simulink model "ley_de_control_no_lineal_MGNLC"  (R2023b)
settings: Solver=VariableStepAuto  StartTime=0.0  StopTime=10.0  FixedStep=1e-5  RelTol=1e-3
values from neighbouring files (symbols this model uses):
  L_d = 6.6    [main.m]    (also in parametros.m = 0.0066)
  L_q = 5.8e-3    (= 0.0058)    [diagrama_polos_y_ceros_LTI.m]    (also in main.m = 5.8; parametros.m; variacion_de_parametros.m)
  P_p = 3    [diagrama_polos_y_ceros_LTI.m]    (also in main.m; parametros.m; variacion_de_parametros.m)
settings Model: Creator=nicol  LastModifiedBy=Julya
settings ModelReferenceCC: ModelReferenceMinAlgLoopOccurrences=on

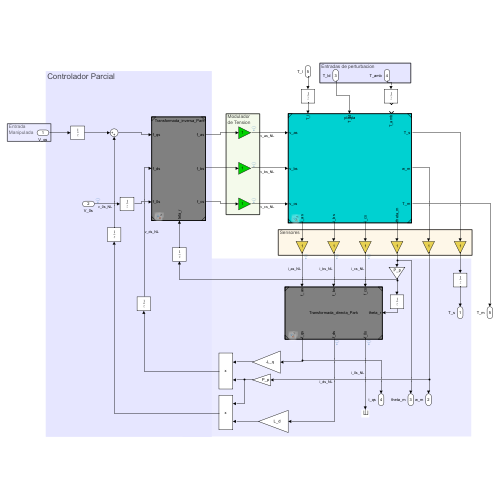
[thumbnail: Simulink's stored preview of the top-level diagram]
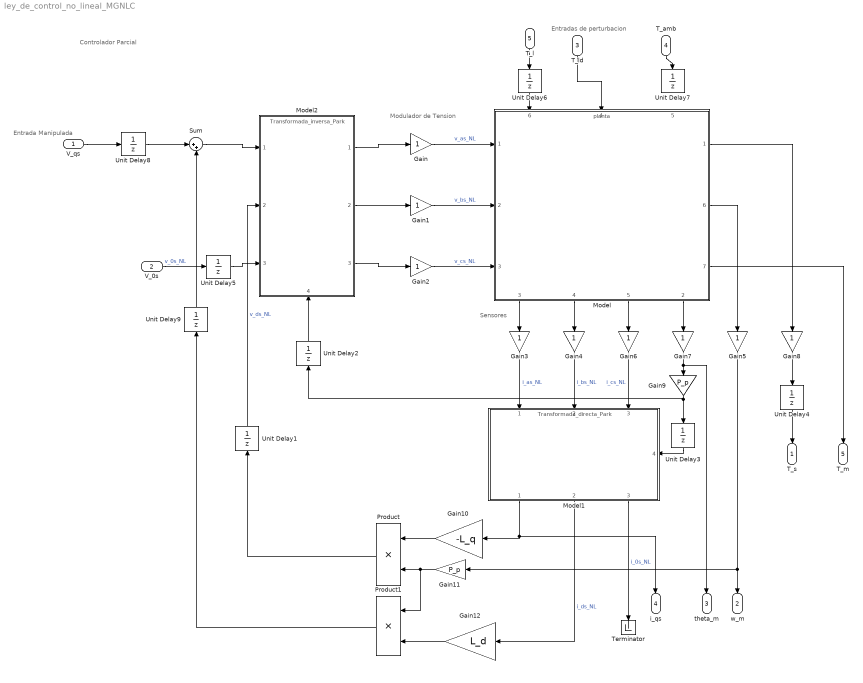
== system ley_de_control_no_lineal_MGNLC ==
  note: Sensores
  note: Modulador
      | de Tension
  note: Entrada
      | Manipulada
  note: Entradas de perturbacion
  note: Controlador Parcial
  V_qs : Inport
  V_0s : Inport  Port=2
  T_ld : Inport  Port=3
  T_amb : Inport  Port=4
  T_l : Inport  Port=5
  Gain{,1..8} (9 alike) : Gain
  Gain10 : Gain  Gain=-L_q
  Gain11 : Gain  Gain=P_p
  Gain12 : Gain  Gain=L_d
  Gain9 : Gain  Gain=P_p
  Model : ModelReference  ModelNameDialog=planta.slx  SimulationMode=Normal  ModelReferenceVersion=1.19
      settings: PortSchema="{\"entries\":[{\"content\":{\"sides\":[{\"content\":{\"connectorIds\":[\"In1\",\"In2\",\"In3\"]},\"type\":\"ConnectorPlacement.EquallySpacedRectSide\",\"uuid\":\"541f2dd0-63a5-498e-b6f4-429df3260999\"},{\"content\":{\"connectorIds\":[\"Out1\",\"Out6\",\"Out7\"],\"side\":\"RIGHT\"},\"type\":\"ConnectorPlacement.EquallySpacedRectSide\",\"uuid\":\"3499a1c9-cb88-4d8d-9b35-501aa0f3df72\"},{\"content\":{\"connectorIds\":[\"In6\",\"In4\",\"In5\"],\"side\":\"TOP\"},\"type\":\"ConnectorPlacement.EquallySpacedRectSide\",\"uuid\":\"c32d79bf-ca05-414a-a73a-795c7b46d2b4\"},{\"content\":{\"connectorIds\":[\"Out3\",\"Out4\",\"Out5\",\"Out2\"],\"side\":\"BOTTOM\"},\"type\":\"ConnectorPlacement.EquallySpacedRectSide\",\"uuid\":\"087f7964-6389-41c1-86e8-9c28c159ac9c\"}]},\"type\":\"ConnectorPlacement.EquallySpacedConnector\",\"uuid\":\"654813cf-572e-4fc9-b0e4-bf7849c76800\"}],\"packageUris\":[\"http://schema.mathworks.com/mf0/Connector/R2020b\"],\"version\":\"1.0\"}"
  Model1 : ModelReference  ModelNameDialog=Transformada_directa_Park.slx  SimulationMode=Normal  ModelReferenceVersion=1.4
      settings: PortSchema="{\"entries\":[{\"content\":{\"sides\":[{\"content\":{\"connectorIds\":[\"In1\",\"In2\",\"In3\"]},\"type\":\"ConnectorPlacement.EquallySpacedRectSide\",\"uuid\":\"82c27493-c118-4c08-95af-31bb68eaa81e\"},{\"content\":{\"connectorIds\":[\"Out1\",\"Out2\",\"Out3\"],\"side\":\"RIGHT\"},\"type\":\"ConnectorPlacement.EquallySpacedRectSide\",\"uuid\":\"a10cc7bc-0b82-4cdd-8936-59a20eab3db5\"},{\"content\":{\"side\":\"TOP\"},\"type\":\"ConnectorPlacement.EquallySpacedRectSide\",\"uuid\":\"5ee0e5c4-eb4f-43d0-8f4c-35007b2184f0\"},{\"content\":{\"connectorIds\":[\"In4\"],\"side\":\"BOTTOM\"},\"type\":\"ConnectorPlacement.EquallySpacedRectSide\",\"uuid\":\"7c6f1f17-2c73-49cd-ba03-ecef4251f566\"}]},\"type\":\"ConnectorPlacement.EquallySpacedConnector\",\"uuid\":\"8bccd47c-0e45-48b8-8fad-d96c8b35cf51\"}],\"packageUris\":[\"http://schema.mathworks.com/mf0/Connector/R2020b\"],\"version\":\"1.0\"}"
  Model2 : ModelReference  ModelNameDialog=Transformada_inversa_Park.slx  SimulationMode=Normal  ModelReferenceVersion=1.5
      settings: PortSchema="{\"entries\":[{\"content\":{\"sides\":[{\"content\":{\"connectorIds\":[\"In1\",\"In2\",\"In3\"]},\"type\":\"ConnectorPlacement.EquallySpacedRectSide\",\"uuid\":\"82c27493-c118-4c08-95af-31bb68eaa81e\"},{\"content\":{\"connectorIds\":[\"Out1\",\"Out2\",\"Out3\"],\"side\":\"RIGHT\"},\"type\":\"ConnectorPlacement.EquallySpacedRectSide\",\"uuid\":\"a10cc7bc-0b82-4cdd-8936-59a20eab3db5\"},{\"content\":{\"side\":\"TOP\"},\"type\":\"ConnectorPlacement.EquallySpacedRectSide\",\"uuid\":\"5ee0e5c4-eb4f-43d0-8f4c-35007b2184f0\"},{\"content\":{\"connectorIds\":[\"In4\"],\"side\":\"BOTTOM\"},\"type\":\"ConnectorPlacement.EquallySpacedRectSide\",\"uuid\":\"7c065461-6f8e-43bc-bbfb-61ddb037de89\"}]},\"type\":\"ConnectorPlacement.EquallySpacedConnector\",\"uuid\":\"8bccd47c-0e45-48b8-8fad-d96c8b35cf51\"}],\"packageUris\":[\"http://schema.mathworks.com/mf0/Connector/R2020b\"],\"version\":\"1.0\"}"
  Product : Product
  Product1 : Product
  Sum : Sum  Inputs=|++
  Terminator : Terminator
  Unit Delay{1..9} (9 alike) : UnitDelay  SampleTime=1e-5  HasFrameUpgradeWarning=on
  T_s : Outport
  w_m : Outport  Port=2
  theta_m : Outport  Port=3
  i_qs : Outport  Port=4
  T_m : Outport  Port=5
  wires:
  Model2/1 -> Gain/1
  Model2/2 -> Gain1/1
  Model2/3 -> Gain2/1
  Gain2/1 -> Model/3  "v_cs_NL"
  Gain1/1 -> Model/2  "v_bs_NL"
  Gain/1 -> Model/1  "v_as_NL"
  Gain4/1 -> Model1/2  "i_bs_NL"
  Model/4 -> Gain4/1
  Model/3 -> Gain3/1
  Gain3/1 -> Model1/1  "i_as_NL"
  Model/5 -> Gain6/1
  Gain6/1 -> Model1/3  "i_cs_NL"
  Model/2 -> Gain7/1
  Model/6 -> Gain5/1
  Model/1 -> Gain8/1
  Gain9/1 -> Unit Delay2/1, Unit Delay3/1
  Gain7/1 -> theta_m/1, Gain9/1
  Gain5/1 -> w_m/1, Gain11/1
  Model1/1 -> i_qs/1, Gain10/1
  Gain11/1 -> Product1/1, Product/2
  Gain10/1 -> Product/1
  Product/1 -> Unit Delay1/1
  V_0s/1 -> Unit Delay5/1  "v_0s_NL"
  T_ld/1 -> Model/4
  Sum/1 -> Model2/1
  Gain12/1 -> Product1/2
  Model1/2 -> Gain12/1  "i_ds_NL"
  Unit Delay1/1 -> Model2/2  "v_ds_NL"
  Unit Delay2/1 -> Model2/4
  Unit Delay3/1 -> Model1/4
  Gain8/1 -> Unit Delay4/1
  T_l/1 -> Unit Delay6/1
  Unit Delay4/1 -> T_s/1
  Unit Delay5/1 -> Model2/3
  Unit Delay6/1 -> Model/6
  T_amb/1 -> Unit Delay7/1
  V_qs/1 -> Unit Delay8/1
  Unit Delay8/1 -> Sum/1
  Model/7 -> T_m/1
  Product1/1 -> Unit Delay9/1
  Unit Delay9/1 -> Sum/2
  Model1/3 -> Terminator/1  "i_0s_NL"
